simulink model "ME419_Ex1_5"  (R2023b)
settings: Solver=VariableStepAuto  StartTime=0.0  StopTime=10.0  RelTol=1e-3
settings Model: Creator=aliawolken  LastModifiedBy=andyjwaideh

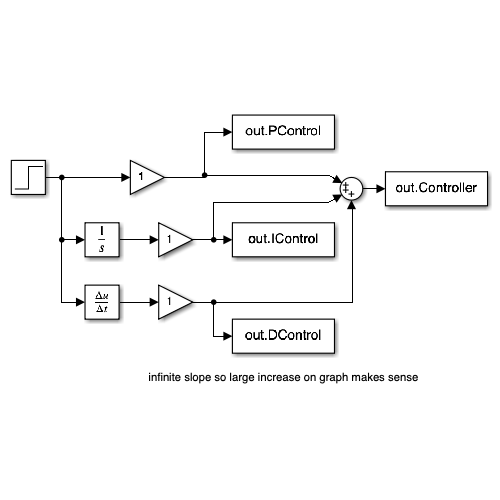
[thumbnail: Simulink's stored preview of the top-level diagram]
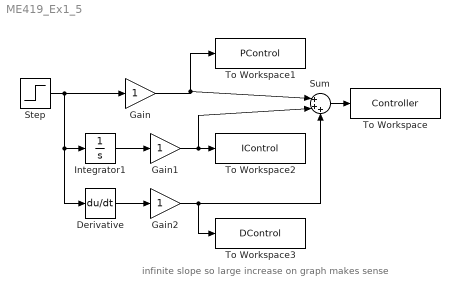
== system ME419_Ex1_5 ==
  note: infinite slope so large increase on graph makes sense
  Derivative : Derivative
  Gain : Gain
  Gain1 : Gain
  Gain2 : Gain
  Integrator1 : Integrator
  Step : Step  SampleTime=0
  Sum : Sum  Inputs=|+++
  To Workspace : ToWorkspace  VariableName=Controller  SampleTime=-1
  To Workspace1 : ToWorkspace  VariableName=PControl  SampleTime=-1
  To Workspace2 : ToWorkspace  VariableName=IControl  SampleTime=-1
  To Workspace3 : ToWorkspace  VariableName=DControl  SampleTime=-1
  wires:
  Gain/1 -> To Workspace1/1, Sum/1
  Integrator1/1 -> Gain1/1
  Gain1/1 -> To Workspace2/1, Sum/2
  Gain2/1 -> Sum/3, To Workspace3/1
  Step/1 -> Gain/1, Derivative/1, Integrator1/1
  Derivative/1 -> Gain2/1
  Sum/1 -> To Workspace/1
